simulink model "modelo"  (R2023a)
settings: Solver=VariableStepAuto  StartTime=0.0  StopTime=25  RelTol=1e-3
model workspace (MAT data in the model file):
  B = 0.00071
  J = 0.00213
  Ke = 0.0921
  Kt = 0.0921
  L = 0.003002923
  R = 2.8614
settings Model: Creator=Alexandre  LastModifiedBy=Alexandre

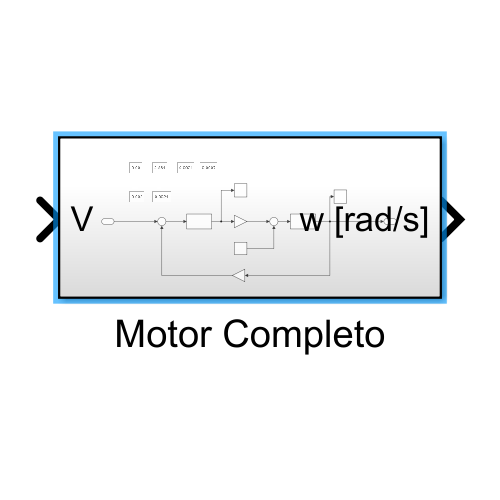
[thumbnail: Simulink's stored preview of the top-level diagram]
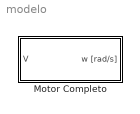
== system modelo ==
  Motor Completo : Subsystem

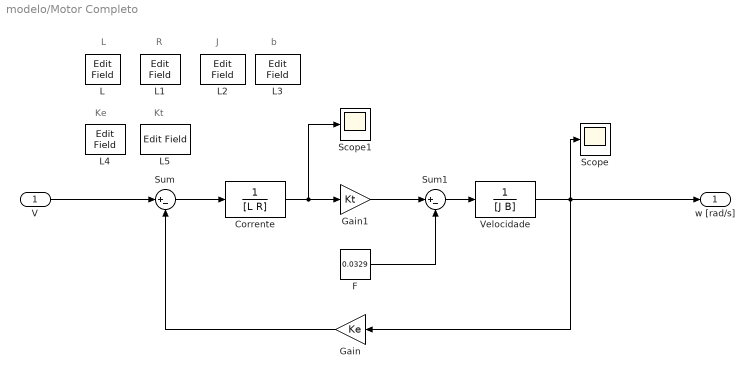
== system modelo/Motor Completo ==
  note: Ke
  note: R
  note: b
  note: J
  note: Kt
  note: L
  V : Inport
  Corrente : TransferFcn  Denominator=[L R]
  F : Constant  Value=0.0329
  Gain : Gain  Gain=Ke
  Gain1 : Gain  Gain=Kt
  L{,1..5} (6 alike) : EditField  LabelPosition=Hide  ShowInitialText=on  Alignment=Center
  Scope : Scope
  Scope1 : Scope
  Sum : Sum  Inputs=|+-
  Sum1 : Sum  Inputs=|+-
  Velocidade : TransferFcn  Denominator=[J B]
  w [rad/s] : Outport
  wires:
  Gain/1 -> Sum/2
  Sum/1 -> Corrente/1
  Sum1/1 -> Velocidade/1
  Gain1/1 -> Sum1/1
  F/1 -> Sum1/2
  Velocidade/1 -> w [rad/s]/1, Scope/1, Gain/1
  Corrente/1 -> Scope1/1, Gain1/1
  V/1 -> Sum/1
